simulink model "Ejemplo7_6_Kuo"  (Simulink 5.0)
settings: Solver=ode45  StartTime=0.0  StopTime=200  RelTol=1e-3
libraries: simulink x1
settings Model: LastModifiedBy=gaby

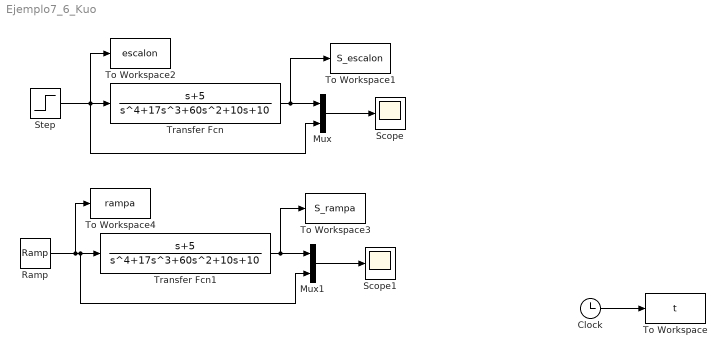
== system Ejemplo7_6_Kuo ==
  Clock : Clock
      settings: Decimation=10
  Mux : Mux  Inputs=2
  Mux1 : Mux  Inputs=2
  Ramp : simulink/Sources/Ramp  slope=1  start=0  X0=0
  Scope : Scope
  Scope1 : Scope
  Step : Step  SampleTime=0
  To Workspace : ToWorkspace  VariableName=t  SampleTime=-1  SaveFormat=Array
  To Workspace1 : ToWorkspace  VariableName=S_escalon  SampleTime=-1  SaveFormat=Array
  To Workspace2 : ToWorkspace  VariableName=escalon  SampleTime=-1  SaveFormat=Array
  To Workspace3 : ToWorkspace  VariableName=S_rampa  SampleTime=-1  SaveFormat=Array
  To Workspace4 : ToWorkspace  VariableName=rampa  SampleTime=-1  SaveFormat=Array
  Transfer Fcn : TransferFcn  Numerator=[1 5]  Denominator=[1 17 60 10 10]
  Transfer Fcn1 : TransferFcn  Numerator=[1 5]  Denominator=[1 17 60 10 10]
  wires:
  Step/1 -> Transfer Fcn/1, Mux/2, To Workspace2/1
  Transfer Fcn/1 -> Mux/1, To Workspace1/1
  Mux/1 -> Scope/1
  Ramp/1 -> Transfer Fcn1/1, Mux1/2, To Workspace4/1
  Transfer Fcn1/1 -> Mux1/1, To Workspace3/1
  Mux1/1 -> Scope1/1
  Clock/1 -> To Workspace/1
